simulink model "Copy_2_of_Driver_Glider"  (R2022b)
settings: Solver=ode45  StartTime=0.0  StopTime=StopTime  FixedStep=1e-4  MaxStep=0.1  RelTol=1e-3  EnableMultiTasking=on
PostLoadFcn:
  | GliderDir = pwd;
  | 
  | cd ..\;
  | SimulinkDir = pwd;
  | addpath(SimulinkDir);
  | 
  | cd(GliderDir);
model workspace (MAT data in the model file):
  DrCycles : object (value not decoded)
  DriverPic = [255 255 255 255 255 255 255 255 255 255 255 255 ... (1049040 elements, 940x372x3)]
  TimeHWFET = 765
  TimeUDDS = 1372
  TimeUS06 = 596
  VehiclePic = [252 252 252 252 252 252 252 252 252 252 252 252 ... (1047540 elements, 316x1105x3)]
  aeroDragCoeff = 0.38
  airDensity = 1.23
  frontArea = 2.1
  gravity = 9.81
  inclinationAngle = 0
  inertialMassVeh = 2392
  massVeh = 2300
  rollingResistCoeff = 0.01
values from neighbouring files (symbols this model uses):
  D_Driver = 0    [Driver_Glider_Params.m]
  GR = Ndriven/Ndriving    (= 12)    [Driver_Glider_Params.m]
  I_Driver = 1    [Driver_Glider_Params.m]
  P_Driver = 7500    [Driver_Glider_Params.m]
  r_wheel = .254    (= 0.254)    [Driver_Glider_Params.m]
  time_step = time(2)    [Driver_Glider_Params.m]
  tractiveForceMax = maxTorque/r_wheel    (= 708.661417323)    [Driver_Glider_Params.m]
undefined symbols (not defined in the file or in its folder): magnitude
libraries: slpidlib x1
(part 2 of 2)

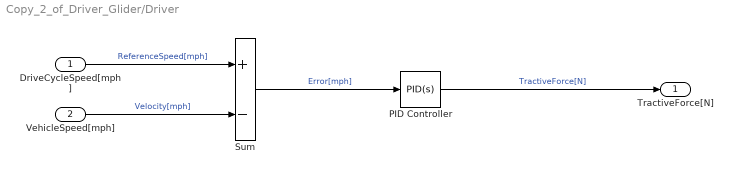
== system Copy_2_of_Driver_Glider/Driver ==
  DriveCycleSpeed[mph] : Inport
  VehicleSpeed[mph] : Inport  Port=2
  PID Controller : slpidlib/PID Controller  Controller=PID  Form=Parallel  TimeDomain=Continuous-time  UseExternalTs=off  SampleTime=-1  IntegratorMethod=Forward Euler  FilterMethod=Forward Euler  ControllerParametersSource=internal  P=P_Driver  I=I_Driver  UseKiTs=off  D=D_Driver  N=100  UseFilter=on  TunerSelectOption=Transfer Function Based (PID Tuner App)  InitialConditionSource=internal  InitialConditionForIntegrator=0  InitialConditionForFilter=0  DifferentiatorICPrevScaledInput=0  ExternalReset=none  TrackingMode=off  Kt=1  LimitOutput=on  SatLimitsSource=internal  UpperSaturationLimit=tractiveForceMax  LowerSaturationLimit=-tractiveForceMax  LinearizeAsGain=on  AntiWindupMode=none  Kb=1  LimitIntegrator=off  UpperIntegratorSaturationLimit=inf  LowerIntegratorSaturationLimit=-inf  POutMin=[]  POutMax=[]  IOutMin=[]  IOutMax=[]  DOutMin=[]  DOutMax=[]  NOutMin=[]  NOutMax=[]  SumOutMin=[]  SumOutMax=[]  SaturationOutMin=[]  SaturationOutMax=[]  PParamMin=[]  PParamMax=[]  IParamMin=[]  IParamMax=[]  DParamMin=[]  DParamMax=[]  NParamMin=[]  NParamMax=[]  KbParamMin=[]  KbParamMax=[]  KtParamMin=[]  KtParamMax=[]  KbOutMin=[]  KbOutMax=[]  KtOutMin=[]  KtOutMax=[]  IntegratorOutMin=[]  IntegratorOutMax=[]  FilterOutMin=[]  FilterOutMax=[]  SumI1OutMin=[]  SumI1OutMax=[]  SumI2OutMin=[]  SumI2OutMax=[]  SumI3OutMin=[]  SumI3OutMax=[]  SumI4OutMin=[]  SumI4OutMax=[]  SumDOutMin=[]  SumDOutMax=[]  DifferentiatorOutMin=[]  DifferentiatorOutMax=[]  FilterDiffOutCoefMin=[]  FilterDiffOutCoefMax=[]  ReciprocalOutMin=[]  ReciprocalOutMax=[]  SumDenOutMin=[]  SumDenOutMax=[]  SumNumOutMin=[]  SumNumOutMax=[]  DivideOutMin=[]  DivideOutMax=[]  UdiffTsProdOutMin=[]  UdiffTsProdOutMax=[]  NTsProdOutMin=[]  NTsProdOutMax=[]  UintegralTsProdOutMin=[]  UintegralTsProdOutMax=[]  UngainTsProdOutMin=[]  UngainTsProdOutMax=[]  ClampingZeroOutDataTypeStr=Inherit: Inherit via back propagation  ClampingZeroOutMin=[]  ClampingZeroOutMax=[]  FilterDenConstantOutDataTypeStr=Inherit: Inherit via back propagation  FilterDenConstantOutMin=[]  FilterDenConstantOutMax=[]  PCopyOutDataTypeStr=Inherit: Inherit via back propagation  PCopyOutMin=[]  PCopyOutMax=[]  NCopyOutDataTypeStr=Inherit: Inherit via back propagation  NCopyOutMin=[]  NCopyOutMax=[]  IntegratorContinuousStateAttributes=''  IntegratorStateMustResolveToSignalObject=off  IntegratorRTWStateStorageClass=Auto  FilterContinuousStateAttributes=''  FilterStateMustResolveToSignalObject=off  FilterRTWStateStorageClass=Auto  ParallelPVariant=InternalParameters  IdealPVariant=Disabled  IVariant=InternalParameters  DVariant=InternalParameters  IntegratorVariant=Continuous  SatVariant=Enabled  AWVariant=Passthrough  PCopyVariant=Disabled  TRVariant=Disabled  FdbkBlocksVariant=Forward  IdealPFdbkVariant=Disabled  SatFdbkVariant=Disabled  DerivativeFilterVariant=ContFilter  NVariant=InternalParameters  NCopyVariant=Disabled  FilterICVariant=InternalICsFilter  IntegratorICVariant=InternalICs  ExternalResetVariant=Disabled  TRSumVariant=Passthrough  SumFdbkVariant=Disabled  SumVariant=Sum_PID  TsampFilterVariant=InternalTs  TsampNgainVariant=Passthrough  TsampIntegralVariant=Passthrough  ExternalSaturationOutDataTypeStr=Inherit: Same as second input
  Sum : Sum  Inputs=+-
  TractiveForce[N] : Outport  VectorParamsAs1DForOutWhenUnconnected=off
  wires:
  DriveCycleSpeed[mph]/1 -> Sum/1  "ReferenceSpeed[mph]"
  Sum/1 -> PID Controller/1  "Error[mph]"
  VehicleSpeed[mph]/1 -> Sum/2  "Velocity[mph]"
  PID Controller/1 -> TractiveForce[N]/1  "TractiveForce[N]"

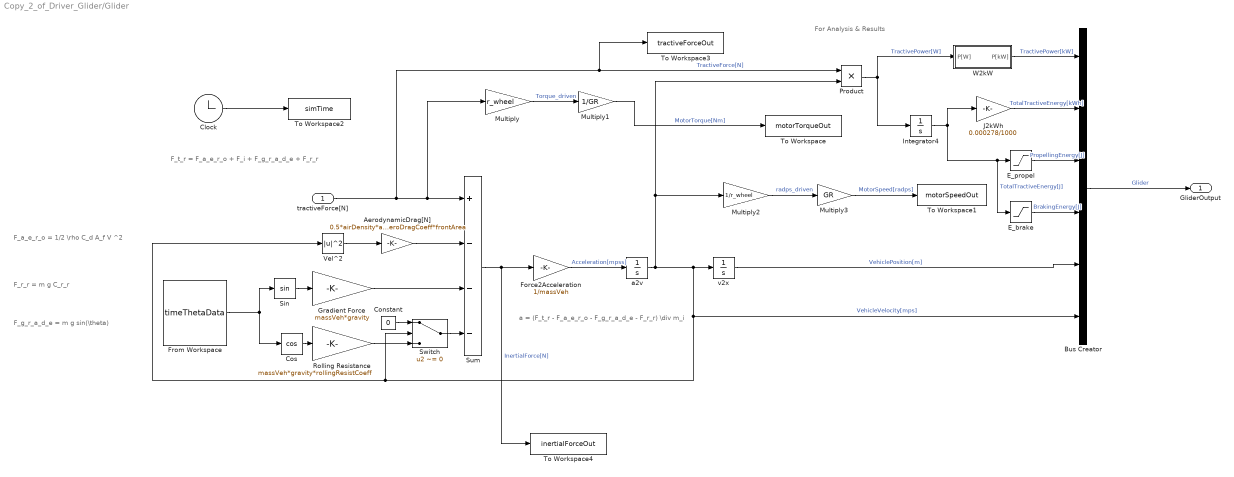
== system Copy_2_of_Driver_Glider/Glider ==
  note: F_t_r = F_a_e_r_o + F_i + F_g_r_a_d_e + F_r_r
  note: a = (F_t_r - F_a_e_r_o - F_g_r_a_d_e - F_r_r) \div m_i
  note: F_r_r = m g C_r_r
  note: For Analysis & Results
  note: F_a_e_r_o = 1/2 \rho C_d A_f V ^2
  note: F_g_r_a_d_e = m g sin(\theta)
  tractiveForce[N] : Inport
  AerodynamicDrag[N] : Gain  Gain=0.5*airDensity*aeroDragCoeff*frontArea
      settings: AttributesFormatString=%<Gain>
  Bus Creator : BusCreator  Inputs=6
  Clock : Clock
  Constant : Constant  Value=0
  Cos : Trigonometry  Operator=cos
  E_brake : Saturate  UpperLimit=0  LowerLimit=-inf
  E_propel : Saturate  UpperLimit=inf  LowerLimit=0
  Force2Acceleration : Gain  Gain=1/massVeh
      settings: AttributesFormatString=%<Gain>
  From Workspace : FromWorkspace  VariableName=timeThetaData  SampleTime=time_step
  Gradient Force : Gain  Gain=massVeh*gravity
  Integrator4 : Integrator
  J2kWh : Gain  Gain=0.000278/1000
  Multiply : Gain  Gain=r_wheel
  Multiply1 : Gain  Gain=1/GR
  Multiply2 : Gain  Gain=1/r_wheel
  Multiply3 : Gain  Gain=GR
  Product : Product
  Rolling Resistance : Gain  Gain=massVeh*gravity*rollingResistCoeff
  Sin : Trigonometry
  Sum : Sum  Inputs=+---
  Switch : Switch  Criteria=u2 ~= 0  SaturateOnIntegerOverflow=off  InputSameDT=off
  To Workspace : ToWorkspace  VariableName=motorTorqueOut  SampleTime=-1
  To Workspace1 : ToWorkspace  VariableName=motorSpeedOut  SampleTime=-1
  To Workspace2 : ToWorkspace  VariableName=simTime  SampleTime=-1
  To Workspace3 : ToWorkspace  VariableName=tractiveForceOut  SampleTime=-1
  To Workspace4 : ToWorkspace  VariableName=inertialForceOut  SampleTime=-1
  Vel^2 : Math  Operator=magnitude^2  SignedPower=on
  W2kW : Subsystem
  a2v : Integrator
  v2x : Integrator
  GliderOutput : Outport  VectorParamsAs1DForOutWhenUnconnected=off
  wires:
  J2kWh/1 -> Bus Creator/2  "TotalTractiveEnergy[kWh]"
  Sum/1 -> To Workspace4/1, Force2Acceleration/1  "InertialForce[N]"
  E_propel/1 -> Bus Creator/3  "PropellingEnergy[J]"
  W2kW/1(P[kW]) -> Bus Creator/1  "TractivePower[kW]"
  Vel^2/1 -> AerodynamicDrag[N]/1
  Integrator4/1 -> E_brake/1, E_propel/1, J2kWh/1  "TotalTractiveEnergy[J]"
  Force2Acceleration/1 -> a2v/1  "Acceleration[mpss]"
  E_brake/1 -> Bus Creator/4  "BrakingEnergy[J]"
  AerodynamicDrag[N]/1 -> Sum/2
  a2v/1 -> Vel^2/1, Switch/2, Bus Creator/6, v2x/1, Multiply2/1, Product/2  "VehicleVelocity[mps]"
  tractiveForce[N]/1 -> To Workspace3/1, Product/1, Multiply/1, Sum/1  "TractiveForce[N]"
  Product/1 -> Integrator4/1, W2kW/1(P[W])  "TractivePower[W]"
  Bus Creator/1 -> GliderOutput/1  "Glider"
  From Workspace/1 -> Sin/1, Cos/1
  Cos/1 -> Rolling Resistance/1
  Sin/1 -> Gradient Force/1
  Multiply/1 -> Multiply1/1  "Torque_driven"
  Multiply2/1 -> Multiply3/1  "radps_driven"
  Multiply3/1 -> To Workspace1/1  "MotorSpeed[radps]"
  Multiply1/1 -> To Workspace/1  "MotorTorque[Nm]"
  v2x/1 -> Bus Creator/5  "VehiclePosition[m]"
  Clock/1 -> To Workspace2/1
  Constant/1 -> Switch/1
  Switch/1 -> Sum/4
  Rolling Resistance/1 -> Switch/3
  Gradient Force/1 -> Sum/3

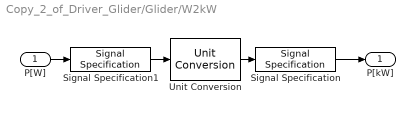
== system Copy_2_of_Driver_Glider/Glider/W2kW ==
  P[W] : Inport
  Signal Specification : SignalSpecification  Unit=kW
  Signal Specification1 : SignalSpecification  Unit=W
  Unit Conversion : UnitConversion
  P[kW] : Outport  VectorParamsAs1DForOutWhenUnconnected=off
  wires:
  Signal Specification/1 -> P[kW]/1
  Signal Specification1/1 -> Unit Conversion/1
  Unit Conversion/1 -> Signal Specification/1
  P[W]/1 -> Signal Specification1/1
